simulink model "release"  (R2021a)
settings: Solver=VariableStepAuto  StartTime=0.0  StopTime=inf  FixedStep=1  RelTol=1e-3
undefined symbols (not defined in the file): f
libraries: instrumentlib x3
settings Model: Creator=花舞  LastModifiedBy=asus
settings SolverCC: AlgebraicLoopSolver=TrustRegion
settings OptimizationCC: OptimizeBlockIOStorage=off  OptimizeDataStoreBuffers=off  BusAssignmentInplaceUpdate=off
settings DebuggingCC: SFUnexpectedBacktrackingDiag=warning  SFNoUnconditionalDefaultTransitionDiag=warning  SFMachineParentedDataDiag=warning
settings RTWCC: GenerateReport=on  BuildConfiguration=Debug  LaunchReport=on
settings CodeAppCC: ForceParamTrailComments=on  MATLABSourceComments=on  EnableCustomComments=on
settings GRTTargetCC: CombineSignalStateStructs=on  SupportVariableSizeSignals=on  MultiInstanceErrorCode=Warning

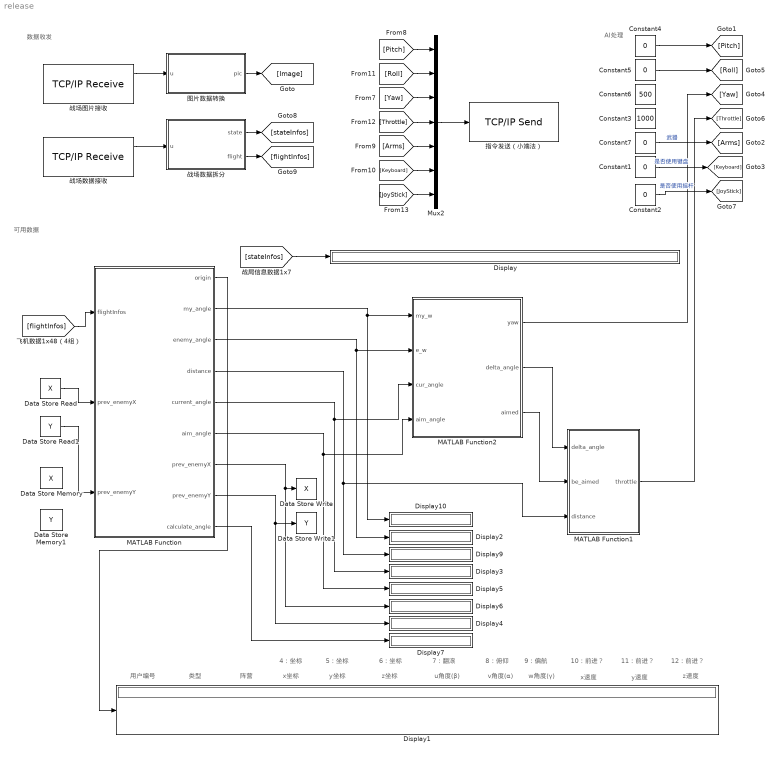
== system release ==
  note: 10：前进？
  note: 4：坐标
  note: 9：偏航
  note: 7：翻滚
  note: 8：俯仰
  note: z速度
  note: y速度
  note: x速度
  note: w角度(γ)
  note: v角度(α)
  note: u角度(β)
  note: z坐标
  note: y坐标
  note: x坐标
  note: 阵营
  note: 类型
  note: 用户编号
  note: AI处理
  note: 可用数据
  note: 数据收发
  note: 5：坐标
  note: 6：坐标
  note: 11：前进？
  note: 12：前进？
  Constant{1..2,4..5,7} (5 alike) : Constant  Value=0  OutDataTypeStr=int32
  Constant3 : Constant  Value=1000  OutDataTypeStr=int32
  Constant6 : Constant  Value=500  OutDataTypeStr=int32
  Data Store Memory : DataStoreMemory  DataStoreName=X  ReadBeforeWriteMsg=warning  WriteAfterWriteMsg=warning  WriteAfterReadMsg=warning  ShowAdditionalParam=off
  Data Store Memory1 : DataStoreMemory  DataStoreName=Y  ReadBeforeWriteMsg=warning  WriteAfterWriteMsg=warning  WriteAfterReadMsg=warning  ShowAdditionalParam=off
  Data Store Read : DataStoreRead  DataStoreName=X  SampleTime=0.1  IndexOptions=Index vector (dialog)  Indices=1  OutputSizes=1
  Data Store Read1 : DataStoreRead  DataStoreName=Y  SampleTime=0.1  IndexOptions=Index vector (dialog)  Indices=1  OutputSizes=1
  Data Store Write : DataStoreWrite  DataStoreName=X  IndexOptions=Index vector (dialog)  Indices=1  OutputSizes=1
  Data Store Write1 : DataStoreWrite  DataStoreName=Y  IndexOptions=Index vector (dialog)  Indices=1  OutputSizes=1
  Display{,1..7,9..10} (10 alike) : Display
  MATLAB Function : MATLAB Function  TreatAsAtomicUnit=on
  MATLAB Function1 : MATLAB Function  TreatAsAtomicUnit=on
  MATLAB Function2 : MATLAB Function  TreatAsAtomicUnit=on
  Mux2 : Mux  Inputs=7
  图片数据转换 : MATLAB Function  TreatAsAtomicUnit=on
  战场图片接收 : instrumentlib/TCP//IP Receive  Host=0.0.0.0  Port=9999  DataSize="[1  1572864]"  EnableBlockingMode=off  Timeout=10  SampleTime=0.01  DataType=uint8  ByteOrder=BigEndian  ASCIIFormatting=%f,  Terminator=LF
  战场数据拆分 : MATLAB Function  TreatAsAtomicUnit=on
  战场数据接收 : instrumentlib/TCP//IP Receive  Host=0.0.0.0  Port=10000  DataSize="[1  55]"  EnableBlockingMode=off  Timeout=10  SampleTime=0.01  DataType=int32  ByteOrder=LittleEndian  ASCIIFormatting=%f,  Terminator=LF
  指令发送（小端法） : instrumentlib/TCP//IP Send  Host=0.0.0.0  Port=9999  EnableBlockingMode=off  Timeout=10  ByteOrder=LittleEndian  TransferDelay=on
  wires:
  Constant7/1 -> [Arms]  "武器"
  Constant1/1 -> [Keyboard]  "是否使用键盘"
  Constant2/1 -> [JoyStick]  "是否使用摇杆"
  [Keyboard] -> Mux2/6
  [Roll] -> Mux2/2
  [Pitch] -> Mux2/1
  [Throttle] -> Mux2/4
  [Yaw] -> Mux2/3
  [Arms] -> Mux2/5
  [JoyStick] -> Mux2/7
  Mux2/1 -> 指令发送（小端法）/1
  [stateInfos] -> Display/1
  [flightInfos] -> MATLAB Function/1(flightInfos)
  战场数据接收/1 -> 战场数据拆分/1(u)
  战场数据拆分/1(state) -> [stateInfos]
  战场数据拆分/2(flight) -> [flightInfos]
  MATLAB Function/1(origin) -> Display1/1
  图片数据转换/1(pic) -> [Image]
  战场图片接收/1 -> 图片数据转换/1(u)
  MATLAB Function/4(distance) -> Display9/1, MATLAB Function1/3(distance)
  MATLAB Function/5(current_angle) -> Display3/1, MATLAB Function2/3(cur_angle)
  Data Store Read/1 -> MATLAB Function/2("prev_enemyX ")
  MATLAB Function/7(prev_enemyX) -> Display6/1, Data Store Write/1
  MATLAB Function/6(aim_angle) -> Display5/1, MATLAB Function2/4(aim_angle)
  Data Store Read1/1 -> MATLAB Function/3("prev_enemyY ")
  MATLAB Function/8(prev_enemyY) -> Display4/1, Data Store Write1/1
  MATLAB Function/2(my_angle) -> Display10/1, MATLAB Function2/1(my_w)
  MATLAB Function/3(enemy_angle) -> Display2/1, MATLAB Function2/2(e_w)
  MATLAB Function2/2(delta_angle) -> MATLAB Function1/1(delta_angle)
  MATLAB Function2/3(aimed) -> MATLAB Function1/2(be_aimed)
  MATLAB Function2/1(yaw) -> [Yaw]
  MATLAB Function1/1(throttle) -> [Throttle]
  Constant5/1 -> [Roll]
  Constant4/1 -> [Pitch]
  MATLAB Function/9(calculate_angle) -> Display7/1

== matlab function release/MATLAB Function ==
  data: origin output; my_angle output; enemy_angle output; distance output; current_angle output; flightInfos input; aim_angle output; prev_enemyX input; prev_enemyX output; prev_enemyY input; prev_enemyY output; calculate_angle output
function [origin,my_angle,enemy_angle,distance,current_angle,aim_angle,prev_enemyX,prev_enemyY,calculate_angle]= data_discrete(flightInfos,prev_enemyX,prev_enemyY)
    origin = flightInfos;
    
    myCoordinate = double(flightInfos(4:6)) / 1000;     % 自己的坐标
    targetCoordinate = double(flightInfos(16:18)) / 1000;     %敌机坐标
    my_x = myCoordinate(1);
    my_y = myCoordinate(2);
    target_x = targetCoordinate(1);%敌机坐标x
    target_y = targetCoordinate(2);%敌机坐标y
    distance = sqrt((target_x - my_x)^2 + (target_y - my_y)^2); %两机距离
    %根据vx和vy计算出来的飞机朝向
    calculate_angle=calculate_v(flightInfos(10),flightInfos(11));
    my_angle = double(flightInfos(9)) / 1000;%传过来的飞机朝向——自己
    enemy_angle = double(flightInfos(21)) / 1000;%传过来的飞机朝向——敌人
    %朝向调整-0.3，根据计算值对比得出
    if my_angle>=0.3
        my_angle=my_angle-0.3;
    else 
        my_angle=my_angle-0.3+2*pi;
    end
    if enemy_angle>=0.3
        enemy_angle=enemy_angle-0.3;
        enemy_angle=enemy_angle -0.3+2*pi;
    end
    
    delta_x = target_x - my_x;
    delta_y = target_y - my_y;
    %计算目标朝向——能瞄准敌机的方向
    angle = acos(delta_x / distance);
    if delta_y >= 0
        current_angle = angle;
    else
        current_angle = 2 * pi - angle;
    end
    
   
    delta_enemyX = target_x - prev_enemyX;
    delta_enemyY = target_y - prev_enemyY;
    delta_distance=sqrt(delta_enemyX^2+delta_enemyY^2);
    if distance <=100
        delta_distance=(0.05+distance/130)*delta_distance;
    end
    predict_enemyX = target_x + delta_distance*cos(enemy_angle);
    predict_enemyY = target_y + delta_distance*sin(enemy_angle);
    
    predict_distance = sqrt((predict_enemyX - my_x)^2 + (predict_enemyY - my_y)^2);
    predict_deltaX= predict_enemyX - my_x;
    predict_deltaY = predict_enemyY - my_y;
    predict_angle = acos(predict_deltaX / predict_distance);
    if predict_deltaY >= 0
        aim_angle = predict_angle;
    else
        aim_angle = 2 * pi - predict_angle;
    end
    % 距离过大时，不用预测值
    if distance >200
        aim_angle=current_angle;
    end
    prev_enemyX = my_x;
    prev_enemyY = my_y;
end



function ret=calculate_v(x,y)
    d =  sqrt(double(x^2 + y^2));
    if y < 0
        ret = 2*pi - acos(double(x/d));
    else
        ret = acos(double(x/d));
    end
end

== matlab function release/战场数据拆分 ==
  data: u input; state output; flight output
function [state,flight] = fcn(u)
state = u(1:7);
flight = u(8:end);

== matlab function release/图片数据转换 ==
  data: u input; pic output
function pic = fcn(u)
coder.extrinsic('image');
col = 1024;
row = 512;
temp = 1;
I = zeros(row, col, 3);
for i=1:row
    for j=1:col
        I(513 - i,j,1)=u(temp);
        I(513 - i,j,2)=u(temp+1);
        I(513 - i,j,3)=u(temp+2);
        temp = temp + 3;
    end
end
pic = double(I)/255;

== matlab function release/MATLAB Function1 ==
  data: delta_angle input; be_aimed input; throttle output; distance input
function throttle = calculate_throttle(delta_angle,be_aimed,distance)
    if be_aimed
        throttle=int32(1000);
    elseif distance <= 50
        throttle=int32(10);
    elseif delta_angle <= pi/3 %距离远，角度近
        throttle=linear(distance);
    elseif delta_angle <=pi/5*3 % 距离远，角度偏大
        throttle=min(linear(distance/2),600);
    else %距离远，相差角度很大
        throttle=int32(300);
    end
end

function ret=linear(t)
    ret=int32(min(1000,t*5));
end

== matlab function release/MATLAB Function2 ==
  data: my_w input; e_w input; cur_angle input; yaw output; aim_angle input; delta_angle output; aimed output
function [yaw,delta_angle,aimed] = calculate_yaw(my_w,e_w,cur_angle,aim_angle)
   aimed = if_aimed(pi*2 - e_w, cur_angle);
   delta_angle = aim_angle - my_w;
    
   % 判断左转还是右转
   sign = -1;
   if delta_angle > 0
       sign = 1;
   end
   delta_angle = abs(delta_angle);
   % 取角度偏小的方向的角度差值,现在的delta_angle取到的区间为[0,pi]
   if delta_angle > pi
       delta_angle =2*pi- delta_angle;
       sign = -sign;  
   end
   
   if aimed
       if delta_angle<pi/4 %角度偏差小于45，角度有点小，可能会撞上敌机，反方向逃离
           delta_angle = pi/3-delta_angle;%15-60偏差
           sign=-sign;
       elseif delta_angle>=pi/4 & delta_angle < pi/2 %说明目前角度在45~90°之间，可以按原来的方向继续走
          delta_angle=0;
       else % 大于90，原定方向偏航，但是delta_angle值减小一点
           delta_angle = delta_angle -45;
       end
   end
   
   if delta_angle < pi/6
       yaw = int32(sign*delta_angle*1000);
   elseif delta_angle >= pi/6 && delta_angle<pi/3
       yaw = int32(sign*delta_angle*800);
   else
       yaw = int32(sign*1000);
   end
end



function flag=if_aimed(angle1,angle2)
    delta=abs(angle1-angle2);
    if delta<=pi/12
        flag=1;
    else
        flag=0;
    end
end
